simulink model "generic_IVS"  (R2024a)
settings: Solver=FixedStepDiscrete  StartTime=0.0  StopTime=inf  FixedStep=0.001  RelTol=1e-3  EnableMultiTasking=on
libraries: CarMaker4SL x57, simulink x1, slpidlib x1
(part 4 of 4)

== matlab function generic_IVS/CarMaker/Subsystem/Final Project/Scenario 1/MATLAB Function ==
  settings: updateMethod=DISCRETE  sampleTime=0.05
  data: waypoints_x input; waypoints_y input; X_ego input; Y_ego input; steering_angle output; speed output; head input; goal_pose input; x_local output; y_local output; GearNo output; is_reverse_path input
function [steering_angle, speed, x_local, y_local, GearNo] = ...
    global_to_local_waypoints(waypoints_x, waypoints_y, ...
                              X_ego, Y_ego, head, goal_pose, is_reverse_path)
%#codegen
    persistent is_reverse_mode goal_point1 debug_counter

    %% 디버깅을 위한 초기화
    if isempty(debug_counter)
        debug_counter = 0;
        goal_point1 = [35, -8];
        is_reverse_mode = false;
    end
    debug_counter = debug_counter + 1;

    %% 1) 파라미터
    stop_threshold          = 4.0;
    heading_align_threshold = 9.0;
    v_base                  = 5.0;   % [m/s]
    v_min                   = 1.5;
    v_max                   = 10.0;
    smooth_window           = 5;     % 웨이포인트 이동평균 윈도우
    alpha_filter            = 0.7;   % 조향각 저역통과 계수 (0~1)

    GearNo = 1;

    %% 2) 유효 웨이포인트 추출 및 스무딩 (중복 제거)
    valid = ~isnan(waypoints_x) & ~isnan(waypoints_y);
    valid_indices = find(valid);  % 유효한 인덱스들 저장
    x_wp0 = waypoints_x(valid);
    y_wp0 = waypoints_y(valid);

    if numel(x_wp0) < 2
        speed = 0; 
        steering_angle = 0;
        x_local = 0;
        y_local = 0;
        GearNo = 1;
        return;
    end

    % 이동평균 스무딩
    x_wp = smoothdata(x_wp0, 'movmean', smooth_window);
    y_wp = smoothdata(y_wp0, 'movmean', smooth_window);

    %% 3) 가장 가까운 포인트 찾기
    dists = hypot(x_wp - X_ego, y_wp - Y_ego);
    [~, idx_closest] = min(dists);

    %% 4) 후진 모드 결정 (수정된 로직 - is_reverse_path 우선 사용)
    % idx_closest는 유효한 웨이포인트 배열의 인덱스이므로 원래 인덱스로 변환
    if idx_closest <= length(valid_indices)
        original_idx = valid_indices(idx_closest);
        % is_reverse_path 배열과 인덱스 매칭하여 후진 모드 결정
        if original_idx <= length(is_reverse_path) && is_reverse_path(original_idx)
            is_reverse_mode = true;
        else
            % 보조적으로 goal_point1 근처 도달 시에도 후진 모드 활성화
            dist_to_goal1 = norm([X_ego - goal_point1(1), Y_ego - goal_point1(2)]);
            if dist_to_goal1 < 4.0
                is_reverse_mode = true;
            end
        end
    end

    %% 5) 로컬 좌표 계산
    dx = x_wp(idx_closest) - X_ego;
    dy = y_wp(idx_closest) - Y_ego;
    x_local = dx*cos(-head) - dy*sin(-head);
    y_local = dx*sin(-head) + dy*cos(-head);

    %% 6) 목표점까지 거리 계산 및 정지/정렬 조건
    goal_dist = norm([X_ego - goal_pose(1), Y_ego - goal_pose(2)]);
    if goal_dist < stop_threshold
        speed = 0; 
        steering_angle = 0; 
        return;
    elseif goal_dist < heading_align_threshold
        heading_error = wrapToPi(pi/2 - head);
        steering_angle = atan2(2*2.9*sin(heading_error), goal_dist + 1e-3);
        speed = 3;
        return;
    end

    %% 7) Pure Pursuit 조향각 계산
    [steer_pp, ~] = pure_pursuit(x_wp, y_wp, [X_ego, Y_ego], head, is_reverse_mode);

    %% 8) 조향각 저역통과 필터
    persistent last_steer
    if isempty(last_steer)
        last_steer = steer_pp;
    end
    steering_angle = alpha_filter * last_steer + (1-alpha_filter) * steer_pp;
    last_steer = steering_angle;

    %% 9) 속도 및 기어 설정
    if is_reverse_mode
        GearNo = -1;
        speed = max(v_min, min(v_max, v_base));  % 양수 속도 유지
    else
        GearNo = 1;
        speed = max(v_min, min(v_max, v_base));   % 양수 속도 (전진)
    end
end

%% ===== Pure Pursuit 함수 =====
function [steering_angle, start_idx] = pure_pursuit(waypoints_x, waypoints_y, vehicle_position, head, is_reverse)
    persistent last_target_idx;
    if isempty(last_target_idx), last_target_idx = 1; end

    WHEEL_BASE = 20.0;
    lookahead_dist = 5.5;
    num_points = length(waypoints_x);

    x_ego = vehicle_position(1);
    y_ego = vehicle_position(2);
    local_waypoints = zeros(num_points, 2);

    % 로컬 좌표 변환
    for i = 1:num_points
        dx = waypoints_x(i) - x_ego;
        dy = waypoints_y(i) - y_ego;
        local_waypoints(i,:) = [ dx*cos(-head)-dy*sin(-head), ...
                                 dx*sin(-head)+dy*cos(-head) ];
    end

    d2 = hypot(waypoints_x - x_ego, waypoints_y - y_ego);
    [~, closest_idx] = min(d2);
    start_idx = max(last_target_idx, closest_idx);

    % 타겟 포인트 선택
    target_idx = -1;
    for i = start_idx:num_points
        if norm(local_waypoints(i,:)) > lookahead_dist
            if (~is_reverse && local_waypoints(i,1) > 0) || ...
               (is_reverse && local_waypoints(i,1) < 0)
                target_idx = i; 
                break;
            end
        end
    end

    % 타겟을 찾지 못한 경우 처음부터 다시 검색
    if target_idx < 0
        for i = 1:start_idx-1
            if norm(local_waypoints(i,:)) > lookahead_dist && local_waypoints(i,1) > 0
                target_idx = i; 
                break;
            end
        end
    end

    if target_idx < 0
        steering_angle = 0; 
        return;
    end

    % Pure Pursuit 알고리즘
    pt = local_waypoints(target_idx,:);
    alpha = wrapToPi(atan2(pt(2), pt(1)));
    ld = min(max(norm(pt), 2.0), 20.0);
    steering_angle = atan2(2*WHEEL_BASE*sin(alpha), ld);

    last_target_idx = target_idx;
end

%% ===== 각도 wrap 함수 =====
function angle = wrapToPi(theta)
    angle = mod(theta + pi, 2*pi) - pi;
end
%% 
% function [steering_angle, speed, x_local, y_local, GearNo] = ...
%     global_to_local_waypoints(waypoints_x, waypoints_y, ...
%                               X_ego, Y_ego, head, goal_pose, is_reverse_path)
% %#codegen
%     persistent is_reverse_mode goal_point1 debug_counter
% 
%     %% 디버깅을 위한 초기화
%     if isempty(debug_counter)
%         debug_counter = 0;
%         goal_point1 = [17, -9];
%         is_reverse_mode = false;
%     end
%     debug_counter = debug_counter + 1;
% 
%     %% 1) 파라미터
%     stop_threshold          = 4.0;
%     heading_align_threshold = 9.0;
%     v_base                  = 5.0;   % [m/s]
%     v_min                   = 1.5;
%     v_max                   = 10.0;
%     smooth_window           = 5;     % 웨이포인트 이동평균 윈도우
%     alpha_filter            = 0.7;   % 조향각 저역통과 계수 (0~1)
% 
%     GearNo = 1;
% 
%     %% 2) 유효 웨이포인트 추출 및 스무딩 (중복 제거)
%     valid = ~isnan(waypoints_x) & ~isnan(waypoints_y);
%     x_wp0 = waypoints_x(valid);
%     y_wp0 = waypoints_y(valid);
%     valid_reverse_path = is_reverse_path(valid);  % 유효한 구간의 후진 정보
% 
%     if numel(x_wp0) < 2
%         speed = 0; 
%         steering_angle = 0;
%         x_local = 0;
%         y_local = 0;
%         GearNo = 1;
%         return;
%     end
% 
%     % 이동평균 스무딩
%     x_wp = smoothdata(x_wp0, 'movmean', smooth_window);
%     y_wp = smoothdata(y_wp0, 'movmean', smooth_window);
% 
%     %% 3) 가장 가까운 포인트 찾기
%     dists = hypot(x_wp - X_ego, y_wp - Y_ego);
%     [~, idx_closest] = min(dists);
% 
%     %% 4) 후진 모드 결정 (개선된 로직)
%     % goal_point1 근처 도달 시 후진 모드 활성화
%     dist_to_goal1 = norm([X_ego - goal_point1(1), Y_ego - goal_point1(2)]);
% 
%     % 후진 모드 전환 조건
%     if dist_to_goal1 < 4.0  % goal_point1 근처 도달
%         is_reverse_mode = true;
%     elseif idx_closest <= numel(valid_reverse_path) && valid_reverse_path(idx_closest)
%         is_reverse_mode = true;
%     end
% 
% 
% 
%     %% 5) 로컬 좌표 계산
%     dx = x_wp(idx_closest) - X_ego;
%     dy = y_wp(idx_closest) - Y_ego;
%     x_local = dx*cos(-head) - dy*sin(-head);
%     y_local = dx*sin(-head) + dy*cos(-head);
% 
%     %% 6) 목표점까지 거리 계산 및 정지/정렬 조건
%     goal_dist = norm([X_ego - goal_pose(1), Y_ego - goal_pose(2)]);
%     if goal_dist < stop_threshold
%         speed = 0; 
%         steering_angle = 0; 
%         return;
%     elseif goal_dist < heading_align_threshold
%         heading_error = wrapToPi(pi/2 - head);
%         steering_angle = atan2(2*2.9*sin(heading_error), goal_dist + 1e-3);
%         speed = 3;
%         return;
%     end
% 
%     %% 7) Pure Pursuit 조향각 계산
%     [steer_pp, ~] = pure_pursuit(x_wp, y_wp, [X_ego, Y_ego], head, is_reverse_mode);
% 
%     %% 8) 조향각 저역통과 필터
%     persistent last_steer
%     if isempty(last_steer)
%         last_steer = steer_pp;
%     end
%     steering_angle = alpha_filter * last_steer + (1-alpha_filter) * steer_pp;
%     last_steer = steering_angle;
% 
%     %% 9) 속도 및 기어 설정
%     if is_reverse_mode
%         GearNo = -1;
%         speed = max(v_min, min(v_max, v_base));  % 음수 속도 (후진)
%     else
%         GearNo = 1;
%         speed = max(v_min, min(v_max, v_base));   % 양수 속도 (전진)
%     end
% end
% 
% %% ===== Pure Pursuit 함수 =====
% function [steering_angle, start_idx] = pure_pursuit(waypoints_x, waypoints_y, vehicle_position, head, is_reverse)
%     persistent last_target_idx;
%     if isempty(last_target_idx), last_target_idx = 1; end
% 
%     WHEEL_BASE = 20.0;
%     lookahead_dist = 5.5;
%     num_points = length(waypoints_x);
% 
%     x_ego = vehicle_position(1);
%     y_ego = vehicle_position(2);
%     local_waypoints = zeros(num_points, 2);
% 
%     % 로컬 좌표 변환
%     for i = 1:num_points
%         dx = waypoints_x(i) - x_ego;
%         dy = waypoints_y(i) - y_ego;
%         local_waypoints(i,:) = [ dx*cos(-head)-dy*sin(-head), ...
%                                  dx*sin(-head)+dy*cos(-head) ];
%     end
% 
%     d2 = hypot(waypoints_x - x_ego, waypoints_y - y_ego);
%     [~, closest_idx] = min(d2);
%     start_idx = max(last_target_idx, closest_idx);
% 
%     % 타겟 포인트 선택
%     target_idx = -1;
%     for i = start_idx:num_points
%         if norm(local_waypoints(i,:)) > lookahead_dist
%             if (~is_reverse && local_waypoints(i,1) > 0) || ...
%                (is_reverse && local_waypoints(i,1) < 0)
%                 target_idx = i; 
%                 break;
%             end
%         end
%     end
% 
%     % 타겟을 찾지 못한 경우 처음부터 다시 검색
%     if target_idx < 0
%         for i = 1:start_idx-1
%             if norm(local_waypoints(i,:)) > lookahead_dist && local_waypoints(i,1) > 0
%                 target_idx = i; 
%                 break;
%             end
%         end
%     end
% 
%     if target_idx < 0
%         steering_angle = 0; 
%         return;
%     end
% 
%     % Pure Pursuit 알고리즘
%     pt = local_waypoints(target_idx,:);
%     alpha = wrapToPi(atan2(pt(2), pt(1)));
%     ld = min(max(norm(pt), 2.0), 20.0);
%     steering_angle = atan2(2*WHEEL_BASE*sin(alpha), ld);
% 
%     last_target_idx = target_idx;
% end
% 
% %% ===== 각도 wrap 함수 =====
% function angle = wrapToPi(theta)
%     angle = mod(theta + pi, 2*pi) - pi;
% end

%%

% function [steering_angle, speed, x_local, y_local, GearNo] = ...
%     global_to_local_waypoints(waypoints_x, waypoints_y, ...
%                               X_ego, Y_ego, head, goal_pose, is_reverse_path)
% %#codegen
%     persistent is_reverse_mode
%     %% 1) 파라미터
%     stop_threshold          = 4.0;
%     heading_align_threshold = 9.0;
%     v_base                  = 5.0;   % [m/s]
%     v_min                   = 1.5;
%     v_max                   = 10.0;
%     smooth_window           = 5;     % 웨이포인트 이동평균 윈도우
%     alpha_filter            = 0.7;   % 조향각 저역통과 계수 (0~1)
% 
%     GearNo = 1;
%     if isempty(is_reverse_mode)
%         is_reverse_mode = false;
%     end
%     valid = ~isnan(waypoints_x) & ~isnan(waypoints_y);
%     x_wp0 = waypoints_x(valid);
%     y_wp0 = waypoints_y(valid);
%     if numel(x_wp0)<2
%         speed = 0; 
%         steering_angle = 0;
%         x_local = 0;
%         y_local = 0;
%         GearNo = 1;
%         return;
%     end
%     x_wp = smoothdata(x_wp0, 'movmean', smooth_window);
%     y_wp = smoothdata(y_wp0, 'movmean', smooth_window);
%     dists = hypot(x_wp - X_ego, y_wp - Y_ego);
%     [~, idx_closest] = min(dists);
% 
%     if is_reverse_path(idx_closest)
%         is_reverse_mode = true;
%     end
% 
%     %% 2) 초기화
%     x_local = 0;  y_local = 0;
%     steering_angle = 0;
%     speed = v_base;
% 
%     %% 3) 목표점까지 거리 계산
%     goal_dist = norm([X_ego - goal_pose(1), Y_ego - goal_pose(2)]);
%     if goal_dist < stop_threshold
%         speed = 0; steering_angle = 0; return;
%     elseif goal_dist < heading_align_threshold
%         heading_error   = wrapToPi(pi/2 - head);
%         steering_angle = atan2(2*2.9*sin(heading_error), goal_dist + 1e-3);
%         speed           = 3;
%         return;
%     end
% 
%     %% 4) 유효 웨이포인트 추출 및 스무딩
%     valid = ~isnan(waypoints_x) & ~isnan(waypoints_y);
%     x_wp0 = waypoints_x(valid);
%     y_wp0 = waypoints_y(valid);
%     if numel(x_wp0)<2
%         speed = 0; return;
%     end
%     % — 이동평균 스무딩 —
%     x_wp = smoothdata(x_wp0, 'movmean', smooth_window);
%     y_wp = smoothdata(y_wp0, 'movmean', smooth_window);
% 
%     %% 5) 가장 가까운 포인트 로컬 좌표
%     dists = hypot(x_wp - X_ego, y_wp - Y_ego);
%     [~, idx_closest] = min(dists);
%     dx = x_wp(idx_closest) - X_ego;
%     dy = y_wp(idx_closest) - Y_ego;
%     x_local = dx*cos(-head) - dy*sin(-head);
%     y_local = dx*sin(-head) + dy*cos(-head);
% 
% 
%     %% 6) Pure Pursuit 조향각 계산
%     [steer_pp, ~] = pure_pursuit(x_wp, y_wp, [X_ego, Y_ego], head, is_reverse_mode);
% 
%     %% 7) 조향각 저역통과 필터
%     persistent last_steer
%     if isempty(last_steer)
%         last_steer = steer_pp;
%     end
%     steering_angle = alpha_filter * last_steer + (1-alpha_filter) * steer_pp;
%     last_steer = steering_angle;
% 
%     %% 8) 속도 제한
%    % speed = max(v_min, min(v_max, v_base));
%    if is_reverse_mode
%         GearNo = -1;
%         speed = max(v_min, min(v_max, v_base));  % 음수 속도
%         %steering_angle = -steering_angle;         % 조향 반전
%    else
%         GearNo = 1;
%         speed = max(v_min, min(v_max, v_base));   % 전진
%     end
% end
% 
% %% ===== Pure Pursuit 함수 (변경 없음) =====
% function [steering_angle, start_idx] = pure_pursuit(waypoints_x, waypoints_y, vehicle_position, head, is_reverse)
%     persistent last_target_idx;
%     if isempty(last_target_idx), last_target_idx = 1; end
% 
%     WHEEL_BASE = 20.0;
%     lookahead_dist = 5.5;
%     num_points = length(waypoints_x);
% 
%     x_ego = vehicle_position(1);
%     y_ego = vehicle_position(2);
%     local_waypoints = zeros(num_points, 2);
% 
%     for i = 1:num_points
%         dx = waypoints_x(i) - x_ego;
%         dy = waypoints_y(i) - y_ego;
%         local_waypoints(i,:) = [ dx*cos(-head)-dy*sin(-head), ...
%                                  dx*sin(-head)+dy*cos(-head) ];
%     end
% 
%     d2 = hypot(waypoints_x - x_ego, waypoints_y - y_ego);
%     [~, closest_idx] = min(d2);
%     start_idx = max(last_target_idx, closest_idx);
% 
%     target_idx = -1;
%     for i = start_idx:num_points
%         if norm(local_waypoints(i,:))>lookahead_dist && ...
%            ((~is_reverse && local_waypoints(i,1)>0) || ...
%             (is_reverse && local_waypoints(i,1)<0))
%             target_idx = i; break;
%         end
%     end
%     if target_idx<0
%         for i = 1:start_idx-1
%             if norm(local_waypoints(i,:))>lookahead_dist && local_waypoints(i,1)>0
%                 target_idx = i; break;
%             end
%         end
%     end
%     if target_idx<0
%         steering_angle = 0; return;
%     end
% 
%     pt = local_waypoints(target_idx,:);
%     alpha = wrapToPi(atan2(pt(2),pt(1)));
%     ld = min(max(norm(pt),2.0),20.0);
%     steering_angle = atan2(2*WHEEL_BASE*sin(alpha), ld);
% 
%     last_target_idx = target_idx;
% end
% 
% %% ===== 각도 wrap 함수 (변경 없음) =====
% function angle = wrapToPi(theta)
%     angle = mod(theta + pi, 2*pi) - pi;
% end

== matlab function generic_IVS/CarMaker/Subsystem/Final Project/Scenario 1/MATLAB Function3 ==
  settings: updateMethod=DISCRETE  sampleTime=0.05
  data: map_boundary input; mapMatrix output size=[1000, 1000]; traffic_info input
%% ======== generate_map_ ======== Ver 2025-05-17 10:40
function mapMatrix  = generate_map_(map_boundary, traffic_info)
    %변수설정
    resolution = 0.05;
    traffic_info_mat = reshape(traffic_info(1:5*21), 5, []).';
    x_values = map_boundary(1:2:end);
    y_values = map_boundary(2:2:end);
    N = size(traffic_info_mat,1);
    x_min = min(x_values);  x_max = max(x_values);
    y_min = min(y_values);  y_max = max(y_values);
    x_size = ceil((x_max-x_min)/resolution);
    y_size = ceil((y_max-y_min)/resolution);
    
    
    mapMatrix = zeros(y_size, x_size); %출력코드
    
    for i = 1:N
        x_c = traffic_info_mat(i, 1);
        y_c = traffic_info_mat(i, 2);
        yaw = traffic_info_mat(i, 3);
        length = traffic_info_mat(i, 4);
        width = traffic_info_mat(i, 5);
        
        if yaw == -1.57079628
            yaw = -pi/2;
        elseif yaw == 1.57079628
            yaw = pi/2;
        end

        dx = length/2;  dy = width/2;
        local = [-dx,-dy; dx,-dy; dx,dy; -dx,dy];
        R = [cos(yaw), -sin(yaw); sin(yaw), cos(yaw)];
        rotated = (R*local')';
        forward_vec = [cos(yaw), sin(yaw)];
        side_vec    = [-sin(yaw), cos(yaw)];
        if yaw == -pi/2
            center = [x_c, y_c] + (length/2)*forward_vec + (width/2)*side_vec;
        else
            center = [x_c, y_c] + (length/2)*forward_vec - (width/2)*side_vec;
        end
        corners = rotated + center;
        x_idx = (corners(:,1)-x_min)/resolution + 1;
        y_idx = (y_max-corners(:,2))/resolution + 1;
        mask = poly2mask(x_idx, y_idx, y_size, x_size);
        mapMatrix(mask) = 1;
    end
end

== matlab function generic_IVS/CarMaker/Subsystem/Final Project/Scenario 1/MATLAB Function4 ==
  settings: updateMethod=DISCRETE  sampleTime=0.05
  data: map input; x_path output; startPose input; goalPose input; y_path output; mapboundary input
function [x_path, y_path] = rrt_star_planner(map, startPose, goalPose, mapboundary)
    %% ===== Persistent 저장 =====
    persistent path_initialized x_path_cached y_path_cached nPath_cached
    maxPathLength = 500;
    resolution    = 0.05;

    if isempty(path_initialized)
        path_initialized = false;
        x_path_cached   = zeros(maxPathLength, 1);
        y_path_cached   = zeros(maxPathLength, 1);
        nPath_cached    = 1;
    end
    if path_initialized
        x_path = x_path_cached(1:nPath_cached);
        y_path = y_path_cached(1:nPath_cached);
        return;
    end
    
    %% 설정
    visualize      = false;
    maxIter        = 5000;
    stepSize       = 2;
    goalSampleRate = 0.1;
    successDistTh  = 15;
    collisionRes   = 0.5;
    searchRadius   = 10;
    safetyDist     = 50;

    %% 바운더리 기반 인덱스 변환용 파라미터
    x_values = mapboundary(1:2:end);
    y_values = mapboundary(2:2:end);
    x_min = min(x_values);
    y_max = max(y_values);

    toGrid = @(x, y) [(x - x_min)/resolution +  1, (y_max - y)/resolution + 1];
    start_grid = toGrid(startPose(1), startPose(2));
    goal_grid  = toGrid(goalPose(1),  goalPose(2));

    %% 트리 초기화
    nodes = struct('x', start_grid(1), 'y', start_grid(2), 'parent', 0, 'cost', 0);
    path   = struct('x', {}, 'y', {}, 'parent', {}, 'cost', {});
    
    %% RRT* 메인 루프
    for iter = 1:maxIter
        if rand < goalSampleRate
            xr = goal_grid;
        else
            xr = [randi([1,size(map,2)]), randi([1,size(map,1)])];
        end

        [nearestIdx, nearXY] = findNearest(nodes, xr);
        theta = atan2(xr(2)-nearXY(2), xr(1)-nearXY(1));
        newXY = nearXY + stepSize * [cos(theta), sin(theta)];

        if isCollision(newXY, map) || ...
           isPathCollision(nearXY, newXY, map, collisionRes) || ...
           isNearObstacle(newXY, map, safetyDist)
            continue;
        end

        nearIdxs = findNearNodes(nodes, newXY, searchRadius);
        minCost   = nodes(nearestIdx).cost + norm(newXY - nearXY);
        minParent = nearestIdx;

        for j = 1:numel(nearIdxs)
            iNode = nearIdxs(j);
            pxy   = [nodes(iNode).x, nodes(iNode).y];
            if ~isPathCollision(pxy, newXY, map, collisionRes)
                c = nodes(iNode).cost + norm(newXY - pxy);
                if c < minCost
                    minCost   = c;
                    minParent = iNode;
                end
            end
        end

        newNode = struct('x', newXY(1), 'y', newXY(2), ...
                         'parent', minParent, 'cost', minCost);
        nodes(end+1) = newNode;
        newIdx       = numel(nodes);

        for j = 1:numel(nearIdxs)
            iNode = nearIdxs(j);
            pxy   = [nodes(iNode).x, nodes(iNode).y];
            c     = newNode.cost + norm([newNode.x,newNode.y] - pxy);
            if c < nodes(iNode).cost && ...
               ~isPathCollision([newNode.x,newNode.y], pxy, map, collisionRes)
                nodes(iNode).parent = newIdx;
                nodes(iNode).cost   = c;
            end
        end

        if visualize
            plot([nodes(newNode.parent).x,newNode.x], ...
                 [nodes(newNode.parent).y,newNode.y], '-r'); hold on;
        end

        if norm(newXY - goal_grid) < successDistTh
            if visualize, disp('[-] GOAL REACHED'); end
            path = backtrace(nodes, newIdx);
            break;
        end
    end

    %% 결과 경로 반환 (인덱스 → 실좌표로 역변환)
    nRaw = min(numel(path), maxPathLength);
    raw_xy = zeros(nRaw,2);
    for k = 1:nRaw
        raw_xy(k,1) = (path(k).x - 1) * resolution + x_min;
        raw_xy(k,2) =  y_max - (path(k).y - 1) * resolution;
    end

    %% === raw_xy만 스무딩 ===
    if nRaw >= 3
        % moving average
        smooth_window = 15;
        xs = movmean(raw_xy(:,1), smooth_window);
        ys = movmean(raw_xy(:,2), smooth_window);
        % 재샘플링
        smoothN = size(raw_xy,1);
        xi = interp1(1:smoothN, xs, linspace(1,smoothN,smoothN), 'linear')';
        yi = interp1(1:smoothN, ys, linspace(1,smoothN,smoothN), 'linear')';
        smooth_xy = [xi, yi];
    else
        smooth_xy = raw_xy;
    end

    %% === Hybrid 직선 구간 추가 ===
    % 파라미터
    pre_steps  = 10;    post_steps = 8;   step_dist = 0.5;
    gx = goalPose(1); gy = goalPose(2);

    % 마지막 RRT* 접점과 그 이전 점으로 방향 구하기
    if size(smooth_xy,1) >= 2
        v = smooth_xy(end,:) - smooth_xy(end-1,:);
    else
        v = goalPose - smooth_xy(end,:);
    end
    v = v / norm(v);                % 단위 벡터
    % 수직 방향 (±90°): [vx;vy] → perp = [ -vy, vx ]
    perp = [-v(2), v(1)];           

    % pre_path: 마지막 지점에서 수직 방향으로 step_dist씩
    pre_path = zeros(pre_steps,2);
    for i = 1:pre_steps
        pre_path(i,:) = smooth_xy(end,:) + perp * (step_dist*i);
    end

    % 목표점 직전 fix point
    mid_pt = pre_path(end,:);

    % post_path: 목표 직후에도 같은 수직 방향 연장
    post_path = zeros(post_steps,2);
    for i = 1:post_steps
        post_path(i,:) = [gx, gy] + perp * (step_dist*i);
    end

    %% === 전체 경로 합치기 ===
    full_path = [ smooth_xy;
                  pre_path;
                  [gx, gy];
                  post_path ];

    %% 캐싱 및 출력
    nFull = min(size(full_path,1), maxPathLength);
    x_path_cached = zeros(maxPathLength,1);
    y_path_cached = zeros(maxPathLength,1);
    x_path_cached(1:nFull) = full_path(1:nFull,1);
    y_path_cached(1:nFull) = full_path(1:nFull,2);
    nPath_cached = nFull;
    path_initialized = true;

    x_path = x_path_cached(1:nFull);
    y_path = y_path_cached(1:nFull);

    % 캐싱
    nFull = size(full_path,1);
    x_path_cached = zeros(maxPathLength,1);
    y_path_cached = zeros(maxPathLength,1);
    x_path_cached(1:nFull) = full_path(:,1);
    y_path_cached(1:nFull) = full_path(:,2);
    nPath_cached = nFull;
    path_initialized = true;

    %% === 부드럽게(Smoothing) ===
    smooth_window = 15;
    if nFull >= smooth_window
        xs = movmean(x_path_cached(1:nFull), smooth_window);
        ys = movmean(y_path_cached(1:nFull), smooth_window);
        smoothN = 100;
        xi = interp1(1:nFull, xs, linspace(1,nFull,smoothN), 'linear')';
        yi = interp1(1:nFull, ys, linspace(1,nFull,smoothN), 'linear')';
        x_path = xi;
        y_path = yi;
    else
        x_path = x_path_cached(1:nFull);
        y_path = y_path_cached(1:nFull);
    end
end

function [idx, xy] = findNearest(nodes, sampleXY)
    d = arrayfun(@(n) hypot(n.x - sampleXY(1), n.y - sampleXY(2)), nodes);
    [~, idx] = min(d);
    xy = [nodes(idx).x, nodes(idx).y];
end

function nearIdxs = findNearNodes(nodes, pos, radius)
    maxNodes = 1000;
    nearIdxs = zeros(1, maxNodes);
    count = 0;
    for i = 1:numel(nodes)
        if hypot(nodes(i).x - pos(1), nodes(i).y - pos(2)) <= radius
            count = count + 1;
            nearIdxs(count) = i;
        end
    end
    nearIdxs = nearIdxs(1:count);
end

function flag = isCollision(pt, map)
    x = round(pt(1)); y = round(pt(2));
    flag = x < 1 || x > size(map,2) || y < 1 || y > size(map,1) || map(y,x) == 1;
end

function flag = isPathCollision(p1, p2, map, step)
    dist = norm(p2 - p1);
    N = max(1, ceil(dist / step));
    flag = false;
    for i = 0:N
        pt = p1 + (p2 - p1) * (i / N);
        if isCollision(pt, map)
            flag = true; return;
        end
    end
end

function flag = isNearObstacle(pt, map, safeDist)
    x0 = round(pt(1)); y0 = round(pt(2));
    r  = ceil(safeDist);
    [X, Y] = meshgrid((x0 - r):(x0 + r), (y0 - r):(y0 + r));
    D2 = (X - pt(1)).^2 + (Y - pt(2)).^2;
    mask = D2 <= safeDist^2;
    X = X(mask); Y = Y(mask);
    valid = X >= 1 & X <= size(map,2) & Y >= 1 & Y <= size(map,1);
    flag  = any(map(sub2ind(size(map), Y(valid), X(valid))) == 1);
end

function path = backtrace(nodes, idx)
    maxPathLen = 500;
    dummyNode = struct('x', 0, 'y', 0, 'parent', 0, 'cost', 0);
    path = repmat(dummyNode, maxPathLen, 1);
    count = 0;
    while idx ~= 0 && count < maxPathLen
        count = count + 1;
        path(count) = nodes(idx);
        idx = nodes(idx).parent;
    end
    path = path(count:-1:1);
end

== matlab function generic_IVS/CarMaker/Subsystem/Final Project/Scenario 1/MATLAB Function6 ==
  data: waypoints_x input; waypoints_y input; steering_angle output; vehicle_position input; head input; start_idx output
% global tracking
function [steering_angle, start_idx] = pure_pursuit(waypoints_x, waypoints_y, vehicle_position, head)

    persistent last_target_idx;
    if isempty(last_target_idx)
        last_target_idx = 1; % 초기값 설정
    end

    WHEEL_BASE = 2.9;

    num_points = length(waypoints_x);

    local_waypoints = zeros(num_points, 2);
    x_ego = vehicle_position(1);
    y_ego = vehicle_position(2);

    for i = 1:num_points
        dx = waypoints_x(i) - x_ego;
        dy = waypoints_y(i) - y_ego;

        local_x = dx * cos(-head) - dy * sin(-head);
        local_y = dx * sin(-head) + dy * cos(-head);

        local_waypoints(i, :) = [local_x, local_y];
    end    

    lookahead_dist = 3.0;

    distances_to_waypoints = sqrt((waypoints_x - x_ego).^2 + (waypoints_y - y_ego).^2);
    [~, closest_idx] = min(distances_to_waypoints);

    start_idx = max(last_target_idx, closest_idx);

    target_idx = -1;
    final_ld = 0;
    for i = start_idx:num_points
        dist = norm(local_waypoints(i, :));
        if dist > lookahead_dist && local_waypoints(i, 1) > 0
            target_idx = i;
            final_ld = dist;
            break;
        end
    end

    if target_idx == -1
        for i = 1:start_idx-1
            dist = norm(local_waypoints(i, :));
            if dist > lookahead_dist && local_waypoints(i, 1) > 0
                target_idx = i;
                final_ld = dist;
                break;
            end
        end
    end

    if target_idx == -1
        steering_angle = 0;
        return;
    end

    target_point = local_waypoints(target_idx, :);
    alpha = atan2(target_point(2), target_point(1));
    alpha = wrapToPi(alpha);

    final_ld = min(max(final_ld, 2.0), 20.0);

    steering_angle = atan2(2 * WHEEL_BASE * sin(alpha), final_ld);

    last_target_idx = target_idx;
end

== stateflow chart generic_IVS/CarMaker/Subsystem/Day3/Chart ==
  (default) -> (junction 1)
  (junction 1) -> (junction 3) [order 1] : [i<99]
      | {i = i + 1;}
  (junction 1) -> (junction 7) [order 2] : {i=0;}
  (junction 3) -> (junction 5)
  (junction 5) -> (junction 7)
  (junction 7) -> (junction 10)
  (junction 10) -> (junction 12) [order 1] : [rem(i,50) == 0]
      | {do_Logic;}
  (junction 10) -> (junction 18) [order 2]
  (junction 12) -> (junction 16)
  (junction 16) -> (junction 18)
  (junction 18) -> (junction 21)
  data: i local =0
  events: do_Logic output FUNCTION_CALL_EVENT
